simulink model "simulink2"  (R2020b)
settings: Solver=VariableStepAuto  StartTime=0.0  StopTime=30  RelTol=1e-3
settings Model: Creator=akku  LastModifiedBy=akku

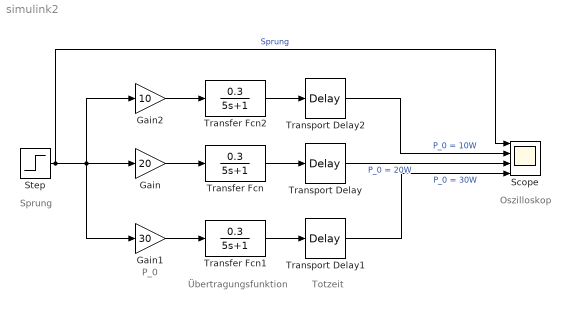
== system simulink2 ==
  note: Oszilloskop
  note: Totzeit
  note: Übertragungsfunktion
  note: P_0
  note: Sprung
  Gain : Gain  Gain=20
  Gain1 : Gain  Gain=30
  Gain2 : Gain  Gain=10
  Scope : Scope  NumInputPorts=4
  Step : Step  Time=0  SampleTime=0
  Transfer Fcn : TransferFcn  Numerator=[0.3]  Denominator=[5 1]
  Transfer Fcn1 : TransferFcn  Numerator=[0.3]  Denominator=[5 1]
  Transfer Fcn2 : TransferFcn  Numerator=[0.3]  Denominator=[5 1]
  Transport Delay : TransportDelay
  Transport Delay1 : TransportDelay
  Transport Delay2 : TransportDelay
  wires:
  Step/1 -> Scope/1, Gain1/1, Gain2/1, Gain/1  "Sprung"
  Transport Delay/1 -> Scope/3  "P_0 = 20W"
  Gain/1 -> Transfer Fcn/1
  Transport Delay2/1 -> Scope/2  "P_0 = 10W"
  Transfer Fcn/1 -> Transport Delay/1
  Gain1/1 -> Transfer Fcn1/1
  Gain2/1 -> Transfer Fcn2/1
  Transfer Fcn1/1 -> Transport Delay1/1
  Transfer Fcn2/1 -> Transport Delay2/1
  Transport Delay1/1 -> Scope/4  "P_0 = 30W"
